simulink model "HSX_current_0214"  (R2023b)
settings: Solver=VariableStepAuto  StartTime=0.0  StopTime=40  RelTol=1e-3
values from neighbouring files (symbols this model uses):
  Iref1 = 8600    [Start.m]
  K1 = OC_K1(1,end)    [Start.m]
  LHSX = 0.02    [Start.m]    (also in Verification.m; cehck.m)
  Ra = 0.0096    [Start.m]    (also in Verification.m; cehck.m)
  RHSX = 0.09    [Start.m]    (also in Verification.m; cehck.m)
  Vf = 0.6    [Start.m]    (also in Verification.m = 4.5; cehck.m = 3.1)
libraries: spsVoltageMeasurementLib x4, spsIdealSwitchLib x3, spsCurrentMeasurementLib x2, spsMosfetLib x2, spsSeriesRLCBranchLib x2, spsDCVoltageSourceLib x1, spsPWMGenerator2LevelLib x1, spsGroundLib x1, spsControlledVoltageSourceLib x1, spsDCMachineLib x1, spsDiodeLib x1, sps_lib x1
settings Model: Creator=Hyeongmeen  LastModifiedBy=Hyeongmeen

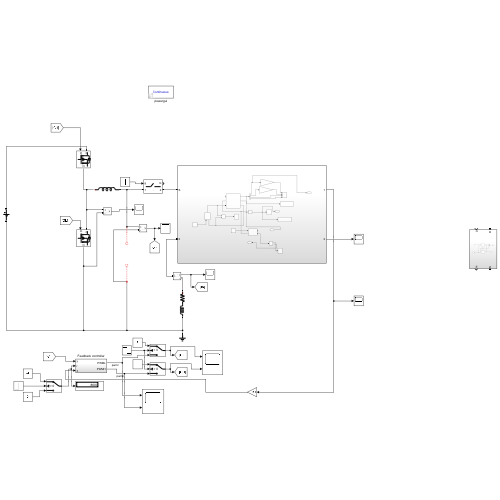
[thumbnail: Simulink's stored preview of the top-level diagram]
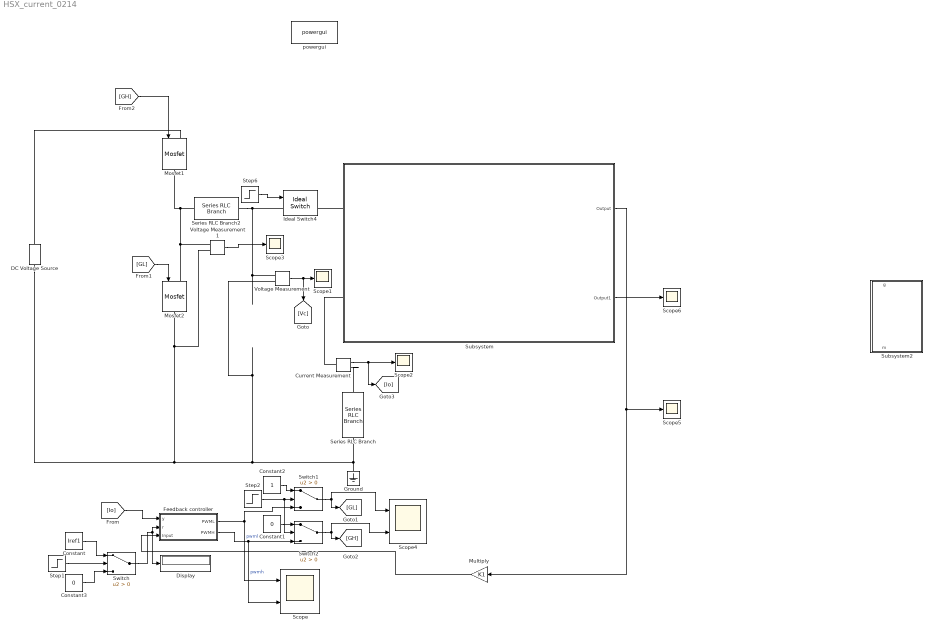
== system HSX_current_0214 ==
  Constant : Constant  Value=Iref1
  Constant1 : Constant  Value=0
  Constant2 : Constant
  Constant3 : Constant  Value=0
  Current Measurement : spsCurrentMeasurementLib/Current Measurement  PhasorSimulation=off  OutputType=Complex  PSBequivalent=0
  DC Voltage Source : spsDCVoltageSourceLib/DC Voltage Source  Amplitude=2400  Measurements=None
  Display : Display
  Feedback controller : Subsystem
  Ground : spsGroundLib/Ground  LConnTagsString=a
  Ideal Switch4 : spsIdealSwitchLib/Ideal Switch  Ron=0  Lon=0  IC=0  Rs=inf  Cs=0  Measurements=on
  Mosfet1 : spsMosfetLib/Mosfet  Ron=0.1  Lon=0  Rd=0.01  Vfd=0.8  IC=0  Rs=1e5  Cs=inf  Measurements=off
  Mosfet2 : spsMosfetLib/Mosfet  Ron=0.1  Lon=0  Rd=0.01  Vfd=0.8  IC=0  Rs=1e5  Cs=inf  Measurements=off
  Multiply : Gain  Gain=K1
  Scope : Scope  NumInputPorts=2
  Scope{1..3,5..6} (5 alike) : Scope
  Scope4 : Scope  NumInputPorts=2
  Series RLC Branch : spsSeriesRLCBranchLib/Series RLC Branch  LConnTagsString=__new0  RConnTagsString=__new0  BranchType=RL  Resistance=RHSX  Inductance=16*LHSX  SetiL0=off  InitialCurrent=0  Capacitance=1e-6  Setx0=off  InitialVoltage=0  Measurements=None
  Series RLC Branch2 : spsSeriesRLCBranchLib/Series RLC Branch  LConnTagsString=__new0  RConnTagsString=__new0  BranchType=L  Resistance=0.09  Inductance=0.0000001  SetiL0=off  InitialCurrent=0  Capacitance=1e-1  Setx0=off  InitialVoltage=0  Measurements=None
  Step1 : Step  Time=21  SampleTime=0  VectorParams1D=off  ZeroCross=off
  Step2 : Step  Time=21  Before=1  After=0  SampleTime=0  VectorParams1D=off  ZeroCross=off
  Step6 : Step  Time=20.1  SampleTime=0  VectorParams1D=off  ZeroCross=off
  Subsystem : Subsystem
  Subsystem2 : Subsystem
  Switch : Switch  Criteria=u2 > Threshold  SaturateOnIntegerOverflow=off  InputSameDT=off
  Switch1 : Switch  Criteria=u2 > Threshold  SaturateOnIntegerOverflow=off  InputSameDT=off
  Switch2 : Switch  Criteria=u2 > Threshold  SaturateOnIntegerOverflow=off  InputSameDT=off
  Voltage Measurement : spsVoltageMeasurementLib/Voltage Measurement  PhasorSimulation=off  OutputType=Complex  PSBequivalent=0
  Voltage Measurement1 : spsVoltageMeasurementLib/Voltage Measurement  PhasorSimulation=off  OutputType=Complex  PSBequivalent=0
  powergui : sps_lib/powergui  Priority=1  SimulationMode=Continuous  SampleTime=1e-7  frequency=60  Iterations=50  frequencyindice=0  Pbase=100e6  ErrMax=1e-4  UnitsV=kV  UnitsW=MW  buscounter=0  FunctionMessages=off  echomessages=off  EnableUseOfTLC=off  CurrentSourceSwitches=off  DisableSnubberDevices=off  DisableRonSwitches=off  DisableVfSwitches=off  DisplayEquations=off  AutomaticDiscreteSolvers=off  SolverType=Tustin/Backward Euler (TBE)  Interpol=off  ExternalGateDelay=off  methode=off  Ts=100  x0status=blocks  SPID=on  SwTol=0  HookPort=off  NonlinearTolerance=1e-4  nMaxIteration=100  ContinueOnMaxIteration=off  RestoreLinks=warning  ResistiveCurrentMeasurement=off  Frange=[0:2:500]  Ylog=off  Xlog=on  ShowGrid=off  save=off  variable=ZData  structure=0  ZoomFFT=off  StartTime=0.0  cycles=1  DisplayStyle=1  fundamental=60  FreqAxis=off  MaxFrequency=1000  frequencyindicesteady=1  RmsSteady=1  display=off
  wires:
  Step6/1 -> Ideal Switch4/1
  Voltage Measurement/1 -> [Vc], Scope1/1
  Current Measurement/1 -> [Io], Scope2/1
  Subsystem/1(Output) -> Scope5/1, Multiply/1
  Switch/1 -> Display/1, Feedback controller/2(r)
  [Io] -> Feedback controller/1(y)
  Feedback controller/1(PWML) -> Switch1/3, Scope/1  "pwml"
  Feedback controller/2(PWMH) -> Switch2/3, Scope/2  "pwmh"
  [GL] -> Mosfet2/1
  Voltage Measurement1/1 -> Scope3/1
  [GH] -> Mosfet1/1
  Step1/1 -> Switch/2
  Constant/1 -> Switch/1
  Switch2/1 -> [GH], Scope4/2
  Switch1/1 -> Scope4/1, [GL]
  Step2/1 -> Switch2/2, Switch1/2
  Constant1/1 -> Switch2/1
  Constant2/1 -> Switch1/1
  Multiply/1 -> Feedback controller/3(Input)
  Constant3/1 -> Switch/3
  Subsystem/2(Output1) -> Scope6/1
  connections:
  Ground/LConn1 -- DC Voltage Source/LConn1 -- Voltage Measurement1/LConn2 -- Mosfet2/RConn1 -- Voltage Measurement/LConn2 -- Series RLC Branch/RConn1
  Ideal Switch4/LConn1 -- Series RLC Branch2/RConn1 -- Voltage Measurement/LConn1
  DC Voltage Source/RConn1 -- Mosfet1/LConn1
  Subsystem/LConn1 -- Ideal Switch4/RConn1
  Current Measurement/LConn1 -- Subsystem/LConn2
  Current Measurement/RConn1 -- Series RLC Branch/LConn1
  Series RLC Branch2/LConn1 -- Voltage Measurement1/LConn1 -- Mosfet2/LConn1 -- Mosfet1/RConn1

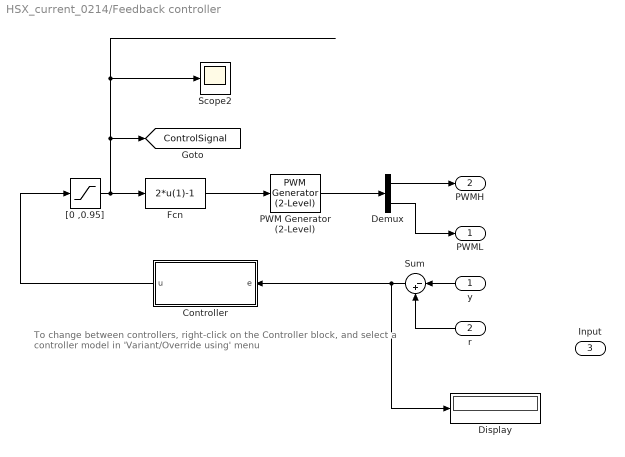
== system HSX_current_0214/Feedback controller ==
  note: To change between controllers, right-click on the Controller block,
      | and select a controller model in 'Variant/Override using' menu
  y : Inport
  r : Inport  Port=2
  Input : Inport  Port=3
  Controller : Subsystem  Variant=on  VariantControlMode=label  LabelModeActiveChoice=Variant1
      settings: AttributesFormatString=%<BlockChoice>
  Demux : Demux  Outputs=2
  Display : Display
  Fcn : Fcn  Expr=2*u(1)-1
  PWM Generator (2-Level) : spsPWMGenerator2LevelLib/PWM Generator (2-Level)  ModulatorType=Single-phase half-bridge (2 pulses)  ModulatorMode=Unsynchronized  Fc=10000  Pc=90  nF=27  MinMax="[ -1  1 ]"  SamplingTechnique=Natural  ModulatingSignals=off  m=0.8  Freq=60  Phase=0  Ts=0  ShowCarrierOutport=off
  Scope2 : Scope
  Sum : Sum  Inputs=|-+  InputSameDT=on  SaturateOnIntegerOverflow=on  OutDataTypeStr=Inherit: Same as first input
  "[0 ,0.95]" : Saturate  UpperLimit=0.95  LowerLimit=0
  PWML : Outport  VectorParamsAs1DForOutWhenUnconnected=off
  PWMH : Outport  Port=2  VectorParamsAs1DForOutWhenUnconnected=off
  tag scope: ControlSignal=global
  wires:
  Controller/1(u) -> "[0 ,0.95]"/1
  Sum/1 -> Controller/1(e), Display/1
  y/1 -> Sum/1
  r/1 -> Sum/2
  "[0 ,0.95]"/1 -> Fcn/1, Scope2/1, [ControlSignal]
  Fcn/1 -> PWM Generator (2-Level)/1
  PWM Generator (2-Level)/1 -> Demux/1
  Demux/1 -> PWMH/1
  Demux/2 -> PWML/1

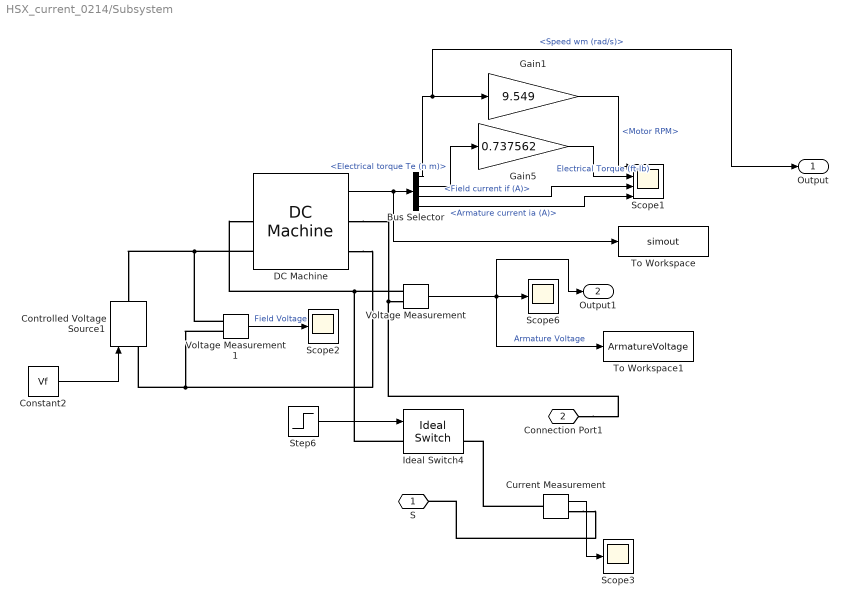
== system HSX_current_0214/Subsystem ==
  Bus Selector : BusSelector  OutputSignals=Speed wm (rad/s),Electrical torque Te (n m),Field current if (A),Armature current ia (A)
  Constant2 : Constant  Value=Vf
  Controlled Voltage Source1 : spsControlledVoltageSourceLib/Controlled Voltage Source  Initialize=on  Source_Type=DC  Amplitude=0  Phase=0  Frequency=0  Measurements=Voltage
  Current Measurement : spsCurrentMeasurementLib/Current Measurement  PhasorSimulation=off  OutputType=Complex  PSBequivalent=0
  DC Machine : spsDCMachineLib/DC Machine  PresetModel=No  MechanicalLoad=Torque TL  FieldType=Wound  ShowDetailedParameters=on  MeasurementBus=off  RLa="[Ra  0.002]"  RLf=[0.0054 0.0125]  Laf=Laf  MachineConstant=Torque constant (N.m/A)  Ke=1.8  Kt=1.8  J=137  Bm=0  Tf=0  w0=w_initial  Ifinit=0  TsPowergui=0  TsBlock=-1
  Gain1 : Gain  Gain=9.549
  Gain5 : Gain  Gain=0.737562
  Ideal Switch4 : spsIdealSwitchLib/Ideal Switch  Ron=0  Lon=0  IC=0  Rs=inf  Cs=0  Measurements=on
  Scope1 : Scope  NumInputPorts=4
  Scope2 : Scope
  Scope3 : Scope
  Scope6 : Scope
  Step6 : Step  Time=20  SampleTime=0  VectorParams1D=off  ZeroCross=off
  To Workspace : ToWorkspace  VariableName=simout  SaveFormat=Timeseries  SampleTime=-1
  To Workspace1 : ToWorkspace  VariableName=ArmatureVoltage  SaveFormat=Timeseries  SampleTime=-1
  Voltage Measurement : spsVoltageMeasurementLib/Voltage Measurement  PhasorSimulation=off  OutputType=Complex  PSBequivalent=0
  Voltage Measurement1 : spsVoltageMeasurementLib/Voltage Measurement  PhasorSimulation=off  OutputType=Complex  PSBequivalent=0
  S : PMIOPort  Side=Left
  Connection Port1 : PMIOPort  Port=2  Side=Left
  Output : Outport
  Output1 : Outport  Port=2
  wires:
  Voltage Measurement/1 -> To Workspace1/1, Scope6/1, Output1/1  "Armature Voltage"
  Voltage Measurement1/1 -> Scope2/1  "Field Voltage"
  Constant2/1 -> Controlled Voltage Source1/1
  Current Measurement/1 -> Scope3/1
  DC Machine/1 -> To Workspace/1, Bus Selector/1
  Gain1/1 -> Scope1/1  "<Motor RPM>"
  Bus Selector/3 -> Scope1/3  "<Field current if (A)>"
  Bus Selector/2 -> Gain5/1  "<Electrical torque Te (n m)>"
  Bus Selector/4 -> Scope1/4  "<Armature current ia (A)>"
  Bus Selector/1 -> Output/1, Gain1/1  "<Speed wm (rad/s)>"
  Gain5/1 -> Scope1/2  "Electrical Torque (ft-lb)"
  Step6/1 -> Ideal Switch4/1
  connections:
  DC Machine/RConn1 -- Connection Port1/RConn1 -- Voltage Measurement/LConn2
  Voltage Measurement/LConn1 -- Ideal Switch4/LConn1 -- DC Machine/LConn1
  DC Machine/LConn2 -- Voltage Measurement1/LConn1 -- Controlled Voltage Source1/RConn1
  DC Machine/RConn2 -- Voltage Measurement1/LConn2 -- Controlled Voltage Source1/LConn1
  Current Measurement/LConn1 -- Ideal Switch4/RConn1
  Current Measurement/RConn1 -- S/RConn1

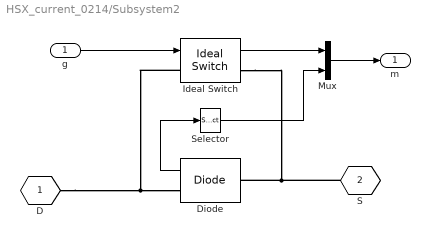
== system HSX_current_0214/Subsystem2 ==
  g : Inport
  Diode : spsDiodeLib/Diode  Ron=1e-3  Lon=0  Vf=Vf  IC=0  UseSnubber=0  Rs=inf  Cs=0  Measurements=on
  Ideal Switch : spsIdealSwitchLib/Ideal Switch  Ron=1e-3  Lon=0  IC=0  Rs=Rs_fet  Cs=Cs_fet  Measurements=on
  Mux : Mux  Inputs=[2,1]
  Selector : Selector  InputPortWidth=2  IndexOptions=Index vector (dialog)  Indices=1  OutputSizes=1
  D : PMIOPort  Tag=PMCPort  Side=Left
  S : PMIOPort  Tag=PMCPort  Port=2  Side=Right
  m : Outport  VectorParamsAs1DForOutWhenUnconnected=off
  wires:
  Ideal Switch/1 -> Mux/1
  Diode/1 -> Selector/1
  Mux/1 -> m/1
  g/1 -> Ideal Switch/1
  Selector/1 -> Mux/2
  connections:
  Ideal Switch/LConn1 -- Diode/RConn1 -- D/RConn1
  Ideal Switch/RConn1 -- Diode/LConn1 -- S/RConn1

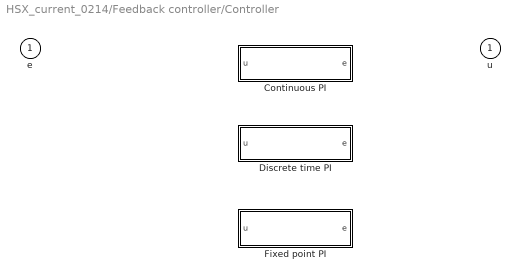
== system HSX_current_0214/Feedback controller/Controller ==
  e : Inport
  Continuous PI : Subsystem  VariantControl=Variant1
  Discrete time PI : Subsystem  VariantControl=Variant2
  Fixed point PI : Subsystem  MinMaxOverflowLogging=MinMaxAndOverflow  VariantControl=Variant3
  u : Outport  VectorParamsAs1DForOutWhenUnconnected=off

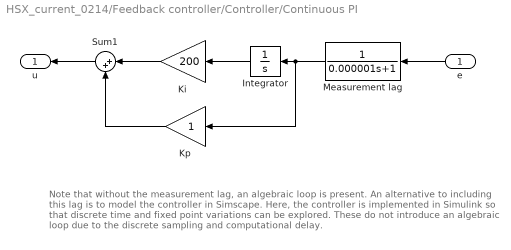
== system HSX_current_0214/Feedback controller/Controller/Continuous PI ==
  note: Note that without the measurement lag, an algebraic loop is present. An alternative to
      | including this lag is to model the controller in Simscape. Here, the controller is implemented
      | in Simulink so that discrete time and fixed point variations can be explored. These do not
      | introduce an algebraic loop due to the discrete sampling and computational delay.
  e : Inport
  Integrator : Integrator
  Ki : Gain  Gain=200
  Kp : Gain
  Measurement lag : TransferFcn  Denominator=[0.000001 1]
  Sum1 : Sum  Inputs=|++  InputSameDT=on  SaturateOnIntegerOverflow=on  OutDataTypeStr=Inherit: Same as first input
  u : Outport  VectorParamsAs1DForOutWhenUnconnected=off
  wires:
  Measurement lag/1 -> Kp/1, Integrator/1
  Ki/1 -> Sum1/1
  Sum1/1 -> u/1
  Kp/1 -> Sum1/2
  Integrator/1 -> Ki/1
  e/1 -> Measurement lag/1

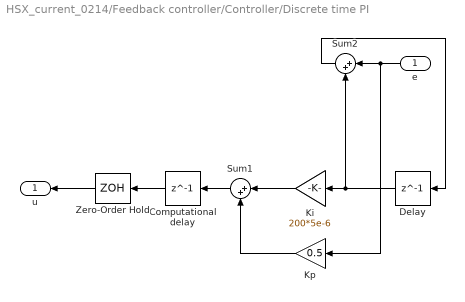
== system HSX_current_0214/Feedback controller/Controller/Discrete time PI ==
  e : Inport
  Computational delay : Delay  DelayLength=1  SampleTime=5e-6
  Delay : Delay  DelayLength=1  SampleTime=5e-6
  Ki : Gain  Gain=200*5e-6
  Kp : Gain  Gain=0.5
  Sum1 : Sum  Inputs=|++  InputSameDT=on  SaturateOnIntegerOverflow=on  OutDataTypeStr=Inherit: Same as first input
  Sum2 : Sum  Inputs=|++  InputSameDT=on  SaturateOnIntegerOverflow=on  OutDataTypeStr=Inherit: Same as first input
  Zero-Order Hold : ZeroOrderHold  SampleTime=5e-6
  u : Outport  VectorParamsAs1DForOutWhenUnconnected=off
  wires:
  Ki/1 -> Sum1/1
  Sum2/1 -> Delay/1
  Delay/1 -> Ki/1, Sum2/2
  Kp/1 -> Sum1/2
  Sum1/1 -> Computational delay/1
  e/1 -> Kp/1, Sum2/1
  Zero-Order Hold/1 -> u/1
  Computational delay/1 -> Zero-Order Hold/1

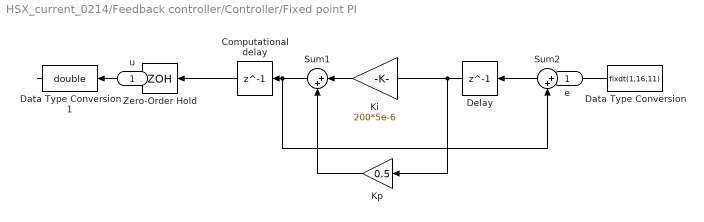
== system HSX_current_0214/Feedback controller/Controller/Fixed point PI ==
  e : Inport
  Computational delay : Delay  DelayLength=1  SampleTime=5e-6
  Data Type Conversion : DataTypeConversion  OutDataTypeStr=fixdt(1,16,11)  RndMeth=Nearest  SaturateOnIntegerOverflow=off
  Data Type Conversion1 : DataTypeConversion  OutDataTypeStr=double  RndMeth=Nearest  SaturateOnIntegerOverflow=off
  Delay : Delay  DelayLength=1  SampleTime=5e-6
  Ki : Gain  Gain=200*5e-6  OutDataTypeStr=fixdt(1,16,13)  RndMeth=Nearest
  Kp : Gain  Gain=0.5  OutDataTypeStr=fixdt(1,16,9)  RndMeth=Nearest
  Sum1 : Sum  Inputs=|++  SaturateOnIntegerOverflow=on
  Sum2 : Sum  Inputs=|++  InputSameDT=on  SaturateOnIntegerOverflow=on  OutDataTypeStr=Inherit: Same as first input
  Zero-Order Hold : ZeroOrderHold  SampleTime=5e-6
  u : Outport  VectorParamsAs1DForOutWhenUnconnected=off
  wires:
  Ki/1 -> Sum1/1
  Data Type Conversion1/1 -> u/1
  Data Type Conversion/1 -> Sum2/1, Kp/1
  Sum1/1 -> Computational delay/1
  Kp/1 -> Sum1/2
  e/1 -> Data Type Conversion/1
  Delay/1 -> Ki/1, Sum2/2
  Sum2/1 -> Delay/1
  Computational delay/1 -> Zero-Order Hold/1
  Zero-Order Hold/1 -> Data Type Conversion1/1
